simulink model "DC_motor"  (R2020a)
settings: Solver=VariableStepAuto  StartTime=0.0  StopTime=10.0  RelTol=1e-3
values from neighbouring files (symbols this model uses):
  b = 3.5077E-6    [DC_MOTOR_DD.sldd]
  J = 3.2284E-6    [DC_MOTOR_DD.sldd]
  k = 0.0274    [DC_MOTOR_DD.sldd]
  kd = 1.0    [DC_MOTOR_DD.sldd]
  ki = 200.0    [DC_MOTOR_DD.sldd]
  kp = 50.0    [DC_MOTOR_DD.sldd]
  L = 2.75E-6    [DC_MOTOR_DD.sldd]
  R = 4.0    [DC_MOTOR_DD.sldd]
settings Model: DataDictionary=DC_MOTOR_DD.sldd  Creator=Admin  LastModifiedBy=Admin
settings DataIOCC: SaveOutput=off  SaveTime=off

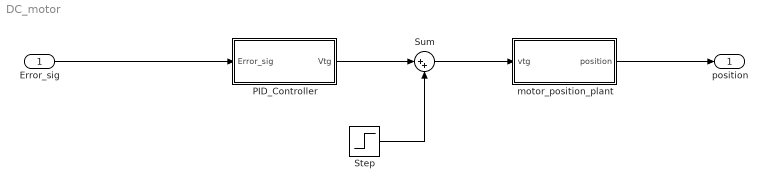
== system DC_motor ==
  Error_sig : Inport  OutDataTypeStr=double  PortDimensions=1  SampleTime=0
  PID_Controller : Subsystem  TreatAsAtomicUnit=on
  Step : Step  Time=0  Before=0.03  SampleTime=0
  Sum : Sum  Inputs=|++
  motor_position_plant : Subsystem  TreatAsAtomicUnit=on
  position : Outport  OutDataTypeStr=double  PortDimensions=1  SampleTime=0
  wires:
  Step/1 -> Sum/2
  PID_Controller/1(Vtg) -> Sum/1
  Sum/1 -> motor_position_plant/1(vtg)
  Error_sig/1 -> PID_Controller/1(Error_sig)
  motor_position_plant/1(position) -> position/1

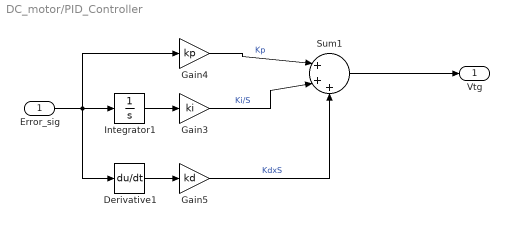
== system DC_motor/PID_Controller ==
  Error_sig : Inport
  Derivative1 : Derivative
  Gain3 : Gain  Gain=ki
  Gain4 : Gain  Gain=kp
  Gain5 : Gain  Gain=kd
  Integrator1 : Integrator
  Sum1 : Sum  Inputs=|+++
  Vtg : Outport
  wires:
  Gain5/1 -> Sum1/3  "KdxS"
  Gain4/1 -> Sum1/1  "Kp"
  Gain3/1 -> Sum1/2  "Ki/S"
  Derivative1/1 -> Gain5/1
  Sum1/1 -> Vtg/1
  Integrator1/1 -> Gain3/1
  Error_sig/1 -> Derivative1/1, Gain4/1, Integrator1/1

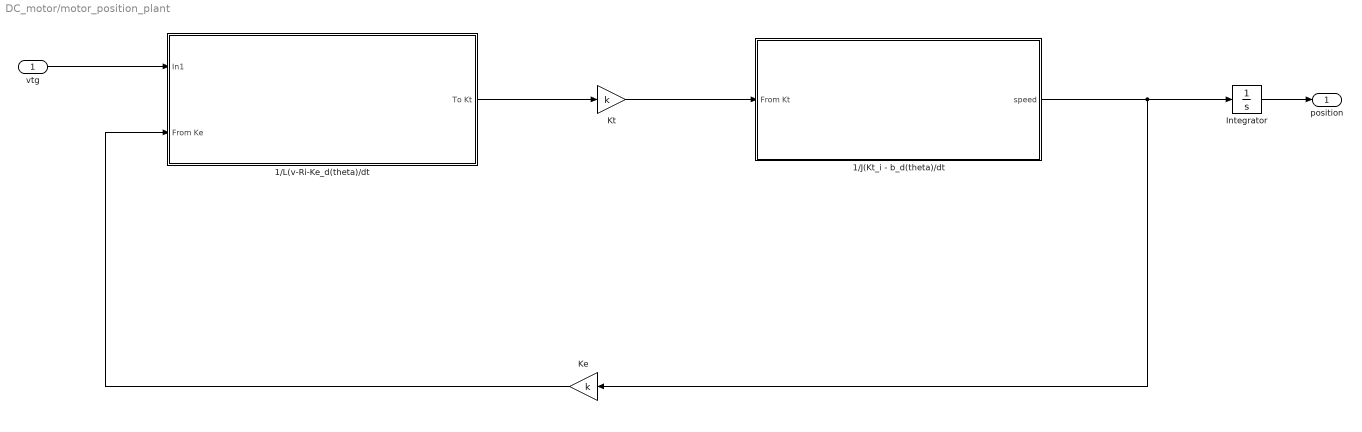
== system DC_motor/motor_position_plant ==
  vtg : Inport
  1/J(Kt_i - b_d(theta)/dt : Subsystem
  1/L(v-Ri-Ke_d(theta)/dt : Subsystem
  Integrator : Integrator
  Ke : Gain  Gain=k
  Kt : Gain  Gain=k
  position : Outport
  wires:
  Ke/1 -> 1/L(v-Ri-Ke_d(theta)/dt/2(From Ke)
  Integrator/1 -> position/1
  1/J(Kt_i - b_d(theta)/dt/1(speed) -> Integrator/1, Ke/1
  1/L(v-Ri-Ke_d(theta)/dt/1(To Kt) -> Kt/1
  Kt/1 -> 1/J(Kt_i - b_d(theta)/dt/1(From Kt)
  vtg/1 -> 1/L(v-Ri-Ke_d(theta)/dt/1(In1)

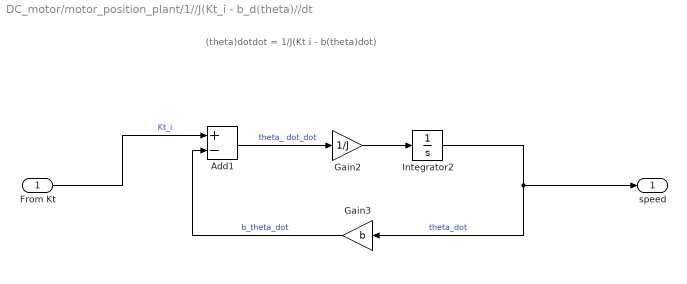
== system DC_motor/motor_position_plant/1//J(Kt_i - b_d(theta)//dt ==
  note: (theta)dotdot = 1/J(Kt i - b(theta)dot)
  From Kt : Inport
  Add1 : Sum  Inputs=+-
  Gain2 : Gain  Gain=1/J
  Gain3 : Gain  Gain=b
  Integrator2 : Integrator
  speed : Outport
  wires:
  Add1/1 -> Gain2/1  "theta_ dot_dot"
  From Kt/1 -> Add1/1  "Kt_i"
  Gain2/1 -> Integrator2/1
  Integrator2/1 -> speed/1, Gain3/1  "theta_dot"
  Gain3/1 -> Add1/2  "b_theta_dot"

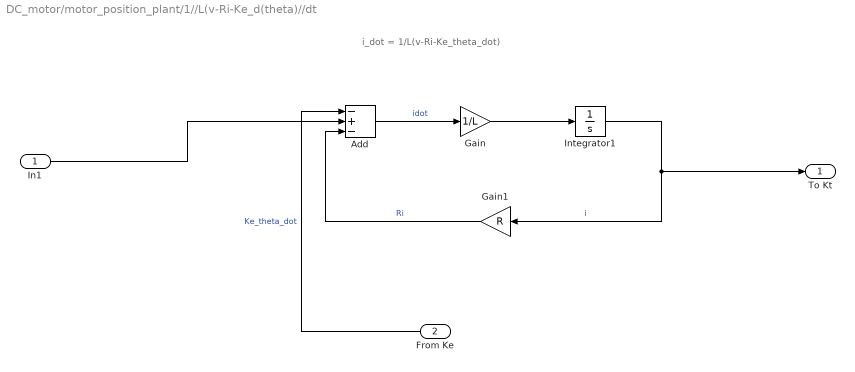
== system DC_motor/motor_position_plant/1//L(v-Ri-Ke_d(theta)//dt ==
  note: i_dot = 1/L(v-Ri-Ke_theta_dot)
  In1 : Inport
  From Ke : Inport  Port=2
  Add : Sum  Inputs=-+-
  Gain : Gain  Gain=1/L
  Gain1 : Gain  Gain=R
  Integrator1 : Integrator
  To Kt : Outport
  wires:
  Gain/1 -> Integrator1/1
  Add/1 -> Gain/1  "idot"
  Integrator1/1 -> To Kt/1, Gain1/1  "i"
  Gain1/1 -> Add/3  "Ri"
  In1/1 -> Add/2
  From Ke/1 -> Add/1  "Ke_theta_dot"
